simulink model "p2_demo_wk1"  (R2024b)
settings: Solver=VariableStepAuto  StartTime=0.0  StopTime=200  RelTol=1e-3
undefined symbols (not defined in the file or in its folder): carData
settings Model: Creator=dxego  LastModifiedBy=swami
settings RTWCC: GPUComputeCapability=3.5

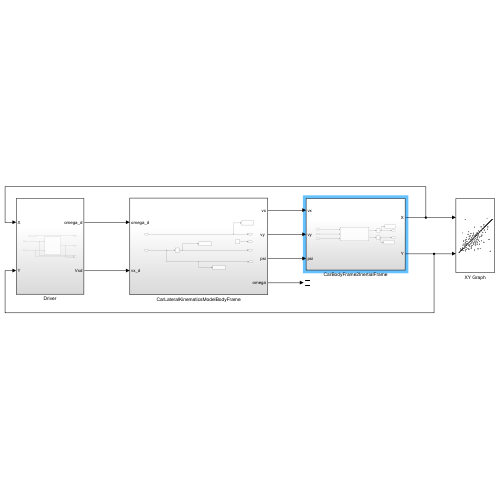
[thumbnail: Simulink's stored preview of the top-level diagram]
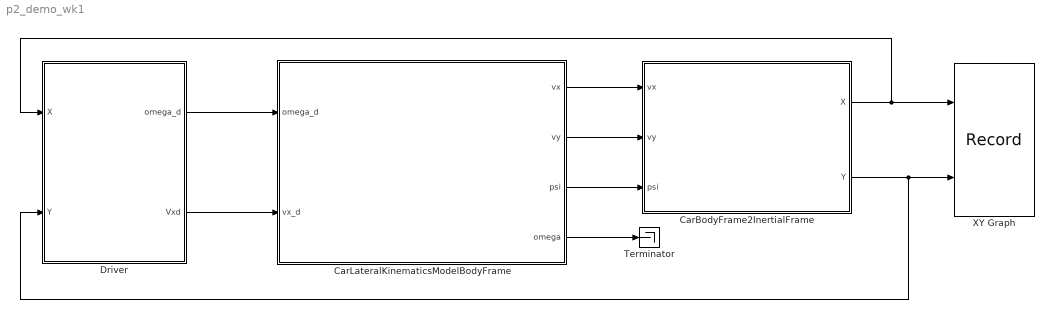
== system p2_demo_wk1 ==
  CarBodyFrame2InertialFrame : Subsystem
  CarLateralKinematicsModelBodyFrame : Subsystem
  Driver : Subsystem
  Terminator : Terminator
  XY Graph : Record  FileSettingsInternal="{\"entries\":[{\"content\":{\"excelSettings\":{\"content\":{},\"type\":\"Streamout.ExcelSettings\"}},\"type\":\"Streamout.FileSettingStorage\",\"uuid\":\"\"}],\"packageUris\":[\"http:\\/\\/schema.mathworks.com\\/mf0\\/streamout_blocks\\/R2020a\"],\"version\":\"1.0\"}"  Layout=[1 1]  SignalsInternal="{\"entries\":[{\"content\":{\"signals\":[{\"content\":{\"blockPath\":[],\"dimensions\":[1],\"domain\":\"\",\"lineColor\":\"#a2142f\",\"plots\":[ 1 ],\"port\":1,\"signalID\":1,\"signalName\":\"CarBodyFrame2InertialFrame:1\"},\"type\":\"RecordBlkView.Signal\",\"uuid\":\"\"},{\"content\":{\"blockPath\":[],\"dimensions\":[1],\"domain\":\"\",\"lineColor\":\"#139fff\",\"plots\":[ 1 ],\"port\":2,\"signalID\":2,\"signalName\":\"CarBodyFrame2InertialFrame:2\"},\"type\":\"RecordBlkView.Signal\",\"uuid\":\"\"}]},\"type\":\"RecordBlkView.InputSignals\",\"uuid\":\"\"}],\"packageUris\":[\"http:\\/\\/schema.mathworks.com\\/mf0\\/streamout_blocks\\/R2020a\"],\"version\":\"1.0\"}"  VisualizationBindings="{\"xyplotplugin\":{\"info\":[{\"series\":[{\"bindingParametersList\":[{\"parameter\":\"X-Axis\",\"signalID\":1,\"signalName\":\"CarBodyFrame2InertialFrame:1\"},{\"parameter\":\"Y-Axis\",\"signalID\":2,\"signalName\":\"CarBodyFrame2InertialFrame:2\"}],\"seriesID\":0}],\"subplotID\":1}]}}"  CompatibilityTag=XY  st=-1
  wires:
  Driver/1(omega_d) -> CarLateralKinematicsModelBodyFrame/1(omega_d)
  CarLateralKinematicsModelBodyFrame/3(psi) -> CarBodyFrame2InertialFrame/3(psi)
  CarBodyFrame2InertialFrame/1(X) -> Driver/1(X), XY Graph/1
  CarBodyFrame2InertialFrame/2(Y) -> Driver/2(Y), XY Graph/2
  Driver/2(Vxd) -> CarLateralKinematicsModelBodyFrame/2("vx_d ")
  CarLateralKinematicsModelBodyFrame/4(omega) -> Terminator/1
  CarLateralKinematicsModelBodyFrame/1(vx) -> CarBodyFrame2InertialFrame/1(vx)
  CarLateralKinematicsModelBodyFrame/2("vy ") -> CarBodyFrame2InertialFrame/2(vy)

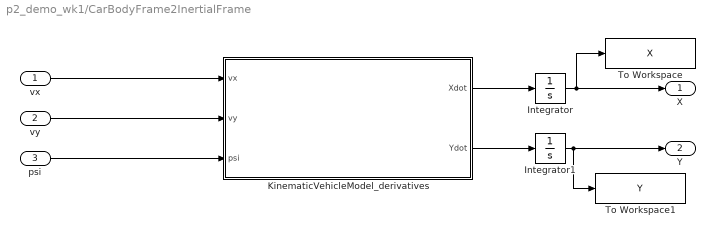
== system p2_demo_wk1/CarBodyFrame2InertialFrame ==
  vx : Inport
  vy : Inport  Port=2
  psi : Inport  Port=3
  Integrator : Integrator  InitialCondition=carData.init.X0
  Integrator1 : Integrator  InitialCondition=carData.init.Y0
  KinematicVehicleModel_derivatives : MATLAB Function  TreatAsAtomicUnit=on
  To Workspace : ToWorkspace  VariableName=X  SaveFormat=Timeseries  SampleTime=-1
  To Workspace1 : ToWorkspace  VariableName=Y  SaveFormat=Timeseries  SampleTime=-1
  X : Outport
  Y : Outport  Port=2
  wires:
  KinematicVehicleModel_derivatives/1(Xdot) -> Integrator/1
  KinematicVehicleModel_derivatives/2(Ydot) -> Integrator1/1
  Integrator/1 -> To Workspace/1, X/1
  Integrator1/1 -> To Workspace1/1, Y/1
  vx/1 -> KinematicVehicleModel_derivatives/1(vx)
  vy/1 -> KinematicVehicleModel_derivatives/2(vy)
  psi/1 -> KinematicVehicleModel_derivatives/3(psi)

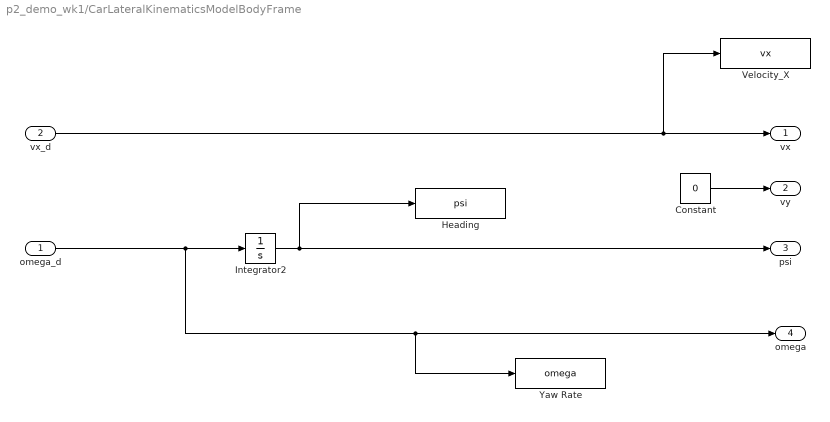
== system p2_demo_wk1/CarLateralKinematicsModelBodyFrame ==
  omega_d : Inport
  "vx_d " : Inport  Port=2
  Constant : Constant  Value=0
  Heading : ToWorkspace  VariableName=psi  SaveFormat=Timeseries  SampleTime=-1
  Integrator2 : Integrator  InitialCondition=carData.init.psi0
  Velocity_X : ToWorkspace  VariableName=vx  SaveFormat=Timeseries  SampleTime=-1
  Yaw Rate : ToWorkspace  VariableName=omega  SaveFormat=Timeseries  SampleTime=-1
  vx : Outport
  "vy " : Outport  Port=2
  psi : Outport  Port=3
  omega : Outport  Port=4
  wires:
  Integrator2/1 -> Heading/1, psi/1
  "vx_d "/1 -> Velocity_X/1, vx/1
  omega_d/1 -> Yaw Rate/1, omega/1, Integrator2/1
  Constant/1 -> "vy "/1

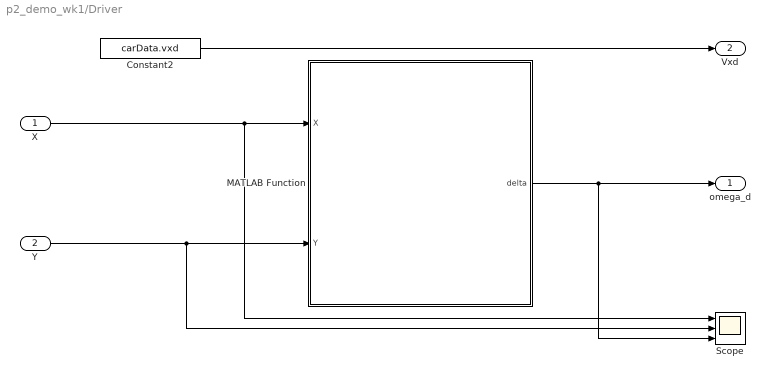
== system p2_demo_wk1/Driver ==
  X : Inport
  Y : Inport  Port=2
  Constant2 : Constant  Value=carData.vxd
  MATLAB Function : MATLAB Function  TreatAsAtomicUnit=on
  Scope : Scope  NumInputPorts=3
  omega_d : Outport
  Vxd : Outport  Port=2
  wires:
  MATLAB Function/1(delta) -> omega_d/1, Scope/3
  Constant2/1 -> Vxd/1
  X/1 -> Scope/1, MATLAB Function/1(X)
  Y/1 -> Scope/2, MATLAB Function/2(Y)

== matlab function p2_demo_wk1/CarBodyFrame2InertialFrame/KinematicVehicleModel_derivatives ==
  data: vx input; vy input; psi input size=1; Xdot output; Ydot output
function [Xdot, Ydot] = fcn(vx, vy, psi)
    temp = TF(psi) * [vx;vy]; 
    Xdot = temp(1);
    Ydot = temp(2);
  
end

function y = TF(psi)
    y = [cos(psi), -sin(psi); sin(psi), cos(psi)];
end

== matlab function p2_demo_wk1/Driver/MATLAB Function ==
  data: X input; delta output; Y input
function delta = SimplestDriver(X,Y)

% %===============================
if abs(Y)<0.5
    delta = 0;
elseif abs(Y - 400) < 0.5
    delta = 0;
elseif X > 900
    delta = 5;
else
    delta = -5;
end



%==============================
% if X > 900
%     delta = .075;
% elseif X < 0
%     delta = -.075;
% else
%     delta = 0;
% end

%===============================
% if X > 900
%     delta = .5;
% elseif X < 0
%     delta = .5;
% else
%     delta = 0;
% end
